simulink model "Modeling"  (R2014a)
settings: Solver=ode45  StartTime=0.0  StopTime=10.0  RelTol=1e-3
settings Model: CovSFcnEnable=on  Creator=Ibrahim  LastModifiedBy=WiZ
settings OptimizationCC: SimCompilerOptimization=off
settings DebuggingCC: MergeDetectMultiDrivingBlocksExec=error  SolverPrmCheckMsg=none  FrameProcessingCompatibilityMsg=error
settings RTWCC: RTWCompilerOptimization=off

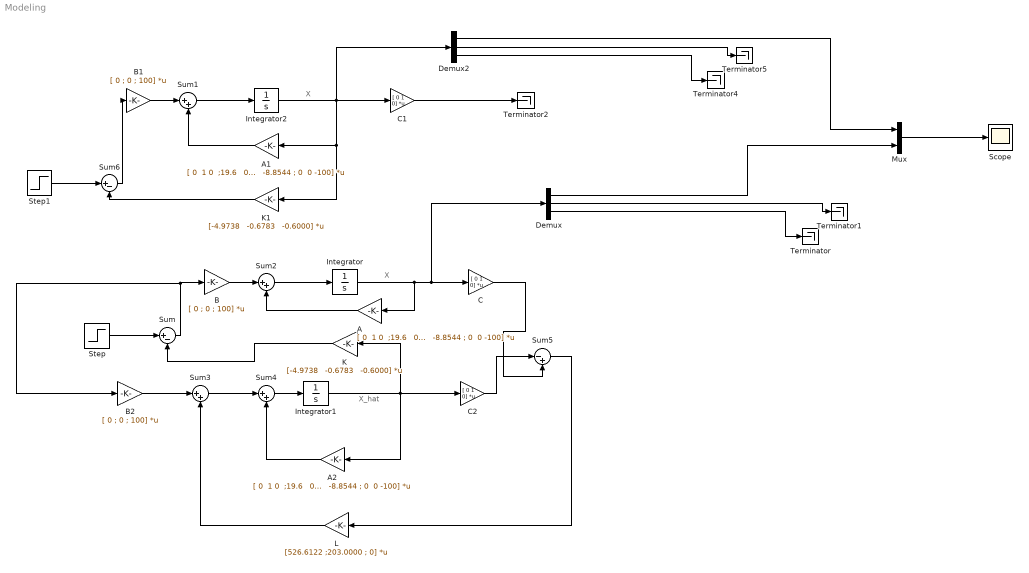
== system Modeling ==
  note: X
  note: X_hat
  note: X
  A : Gain  Gain=|  Multiplication=Matrix(K*u)
      | [ 0  1 0  ;19.6   0   -8.8544
      | ; 0  0 -100]
  A1 : Gain  Gain=|  Multiplication=Matrix(K*u)
      | [ 0  1 0  ;19.6   0   -8.8544
      | ; 0  0 -100]
  A2 : Gain  Gain=|  Multiplication=Matrix(K*u)
      | [ 0  1 0  ;19.6   0   -8.8544
      | ; 0  0 -100]
  B : Gain  Gain=|  Multiplication=Matrix(K*u)
      | [ 0
      | ; 0
      | ; 100]
  B1 : Gain  Gain=|  Multiplication=Matrix(K*u)
      | [ 0
      | ; 0
      | ; 100]
  B2 : Gain  Gain=|  Multiplication=Matrix(K*u)
      | [ 0
      | ; 0
      | ; 100]
  C : Gain  Gain="[ 0     1     0]"  Multiplication=Matrix(K*u)
  C1 : Gain  Gain="[ 0     1     0]"  Multiplication=Matrix(K*u)
  C2 : Gain  Gain="[ 0     1     0]"  Multiplication=Matrix(K*u)
  Demux : Demux  Outputs=3
  Demux2 : Demux  Outputs=3
  Integrator : Integrator  InitialCondition=[0.05;0.05;0.05]
  Integrator1 : Integrator  InitialCondition=[0.15;0.15;0.15]
  Integrator2 : Integrator  InitialCondition=[0.05;0.05;0.05]
  K : Gain  Gain="[-4.9738   -0.6783   -0.6000]"  Multiplication=Matrix(K*u)
  K1 : Gain  Gain="[-4.9738   -0.6783   -0.6000]"  Multiplication=Matrix(K*u)
  L : Gain  Gain=|  Multiplication=Matrix(K*u) (u vector)
      | [526.6122
      | ;203.0000
      | ; 0]
  Mux : Mux  Inputs=2
  Scope : Scope
      settings: YMin=-0.00625017  YMax=0.05625
  Step : Step  Time=0  After=0  SampleTime=0
  Step1 : Step  Time=0  After=0  SampleTime=0
  Sum : Sum  Inputs=|+-
  Sum{1..4} (4 alike) : Sum  Inputs=|++
  Sum5 : Sum  Inputs=|-+
  Sum6 : Sum  Inputs=|+-
  Terminator{,1..2,4..5} (5 alike) : Terminator
  wires:
  Step/1 -> Sum/1
  B/1 -> Sum2/1
  Sum2/1 -> Integrator/1
  A/1 -> Sum2/2
  K/1 -> Sum/2
  Sum/1 -> B/1, B2/1
  Sum4/1 -> Integrator1/1
  A2/1 -> Sum4/2
  L/1 -> Sum3/2
  B2/1 -> Sum3/1
  Sum3/1 -> Sum4/1
  C2/1 -> Sum5/1
  C/1 -> Sum5/2
  Demux/3 -> Terminator/1
  Demux/2 -> Terminator1/1
  Mux/1 -> Scope/1
  Integrator/1 -> Demux/1, C/1, A/1
  Integrator1/1 -> K/1, A2/1, C2/1
  Sum5/1 -> L/1
  Demux/1 -> Mux/2
  B1/1 -> Sum1/1
  Sum1/1 -> Integrator2/1
  A1/1 -> Sum1/2
  Sum6/1 -> B1/1
  Step1/1 -> Sum6/1
  Integrator2/1 -> K1/1, A1/1, Demux2/1, C1/1
  K1/1 -> Sum6/2
  Demux2/3 -> Terminator4/1
  Demux2/2 -> Terminator5/1
  Demux2/1 -> Mux/1
  C1/1 -> Terminator2/1
